simulink model "rw_controller"  (R2024a)
settings: Solver=ode45  StartTime=0.0  StopTime=1000  FixedStep=1E-4  RelTol=1e-3
values from neighbouring files (symbols this model uses):
  gamma_p = 0.1    [simulationParameters.m]    (also in untitled10.m)
  Kp_init = 1    [simulationParameters.m]    (also in untitled10.m)
undefined symbols (not defined in the file or in its folder): init, motor
settings Model: Creator=b_ant  LastModifiedBy=b_ant
settings DataIOCC: SaveFormat=Array

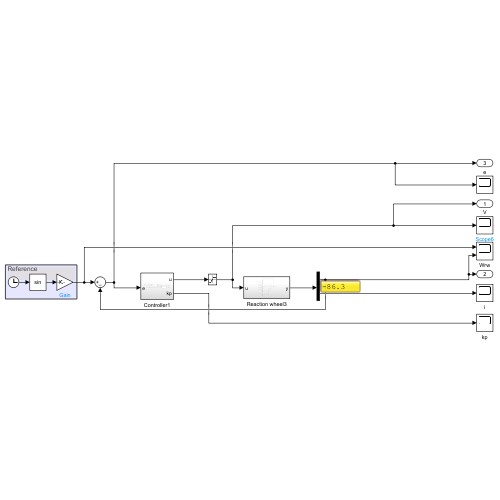
[thumbnail: Simulink's stored preview of the top-level diagram]
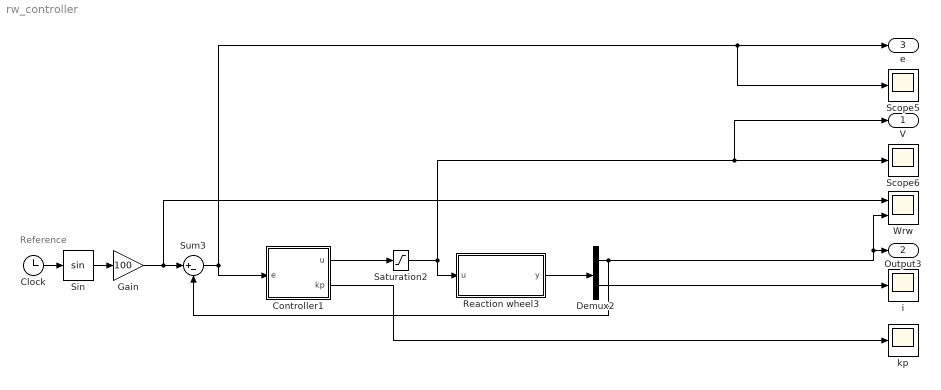
== system rw_controller ==
  note: Reference
  Clock : Clock
  Controller1 : Subsystem
  Demux2 : Demux  Outputs=2
  Gain : Gain  Gain=100
  Reaction wheel3 : Subsystem
  Saturation2 : Saturate  UpperLimit=12  LowerLimit=-12
  Scope5 : Scope
  Scope6 : Scope
  Sin : Trigonometry
  Sum3 : Sum  Inputs=|+-
  Wrw : Scope  NumInputPorts=2
  i : Scope
  kp : Scope
  V : Outport
  Output3 : Outport  Port=2
  e : Outport  Port=3
  wires:
  Sum3/1 -> Controller1/1(e), Scope5/1, e/1
  Reaction wheel3/1(y) -> Demux2/1
  Controller1/1(u) -> Saturation2/1
  Demux2/2 -> i/1
  Saturation2/1 -> Reaction wheel3/1(u), V/1, Scope6/1
  Demux2/1 -> Wrw/2, Output3/1, Sum3/2
  Gain/1 -> Sum3/1, Wrw/1
  Clock/1 -> Sin/1
  Sin/1 -> Gain/1
  Controller1/2(kp) -> kp/1

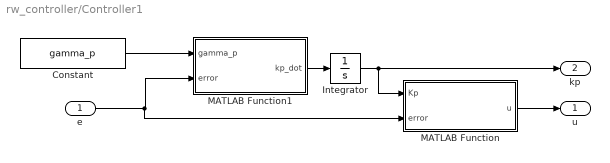
== system rw_controller/Controller1 ==
  e : Inport
  Constant : Constant  Value=gamma_p
  Integrator : Integrator  InitialCondition=Kp_init
  MATLAB Function : MATLAB Function  TreatAsAtomicUnit=on
  MATLAB Function1 : MATLAB Function  TreatAsAtomicUnit=on
  u : Outport
  kp : Outport  Port=2
  wires:
  MATLAB Function/1(u) -> u/1
  MATLAB Function1/1(kp_dot) -> Integrator/1
  Integrator/1 -> kp/1, MATLAB Function/1(Kp)
  e/1 -> MATLAB Function/2(error), MATLAB Function1/2(error)
  Constant/1 -> MATLAB Function1/1(gamma_p)

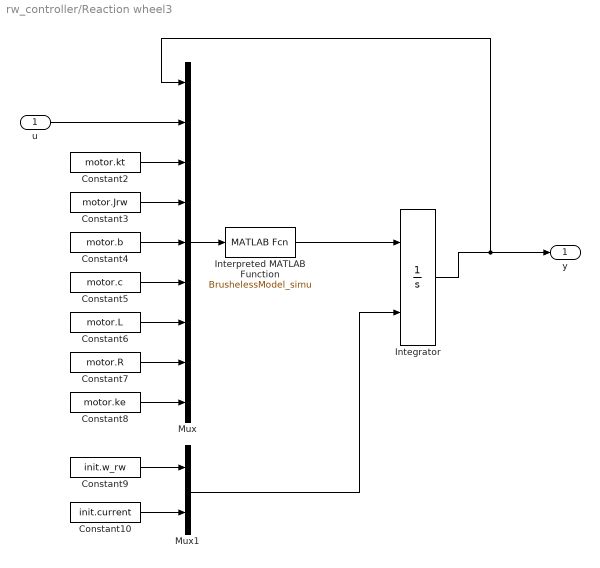
== system rw_controller/Reaction wheel3 ==
  u : Inport
  Constant10 : Constant  Value=init.current
  Constant2 : Constant  Value=motor.kt
  Constant3 : Constant  Value=motor.Jrw
  Constant4 : Constant  Value=motor.b
  Constant5 : Constant  Value=motor.c
  Constant6 : Constant  Value=motor.L
  Constant7 : Constant  Value=motor.R
  Constant8 : Constant  Value=motor.ke
  Constant9 : Constant  Value=init.w_rw
  Integrator : Integrator  InitialConditionSource=external
  Interpreted MATLAB Function : MATLABFcn  MATLABFcn=BrushelessModel_simu  OutputDimensions=2
  Mux : Mux  Inputs=9
  Mux1 : Mux  Inputs=2
  y : Outport
  wires:
  Interpreted MATLAB Function/1 -> Integrator/1
  Constant8/1 -> Mux/9
  Integrator/1 -> Mux/1, y/1
  Constant10/1 -> Mux1/2
  Constant9/1 -> Mux1/1
  Mux/1 -> Interpreted MATLAB Function/1
  Mux1/1 -> Integrator/2
  u/1 -> Mux/2
  Constant2/1 -> Mux/3
  Constant3/1 -> Mux/4
  Constant4/1 -> Mux/5
  Constant5/1 -> Mux/6
  Constant6/1 -> Mux/7
  Constant7/1 -> Mux/8

== matlab function rw_controller/Controller1/MATLAB Function ==
  data: Kp input; u output; error input
function u = P_control(Kp,error)
    u = Kp * error;
end

== matlab function rw_controller/Controller1/MATLAB Function1 ==
  data: gamma_p input; kp_dot output; error input
function kp_dot = fcn(gamma_p,error)
    kp_dot = gamma_p * abs(error);
end
